simulink model "Intro2AV_FinalProjectModel_DT"  (R2024b)
settings: Solver=VariableStepAuto  StartTime=0.0  StopTime=72  RelTol=1e-3
values from neighbouring files (symbols this model uses):
  gradbp = linspace(0,totalDistance,50)    [scriptRefDataDT.m]
  thetaRefs = smooth(gradbp,thetaRef)    [scriptRefDataDT.m]
  xRef2s = smooth(gradbp,xRef2)    [scriptRefDataDT.m]
  yRef2s = smooth(gradbp,yRef2)    [scriptRefDataDT.m]
libraries: drivingvehiclecontroller x1
settings Model: Creator=lpdtd  LastModifiedBy=lpdtd

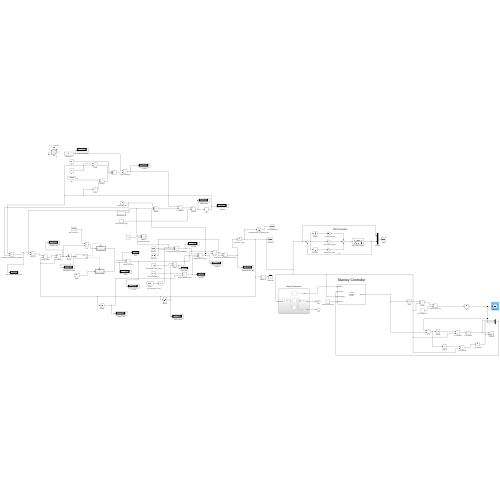
[thumbnail: Simulink's stored preview of the top-level diagram]
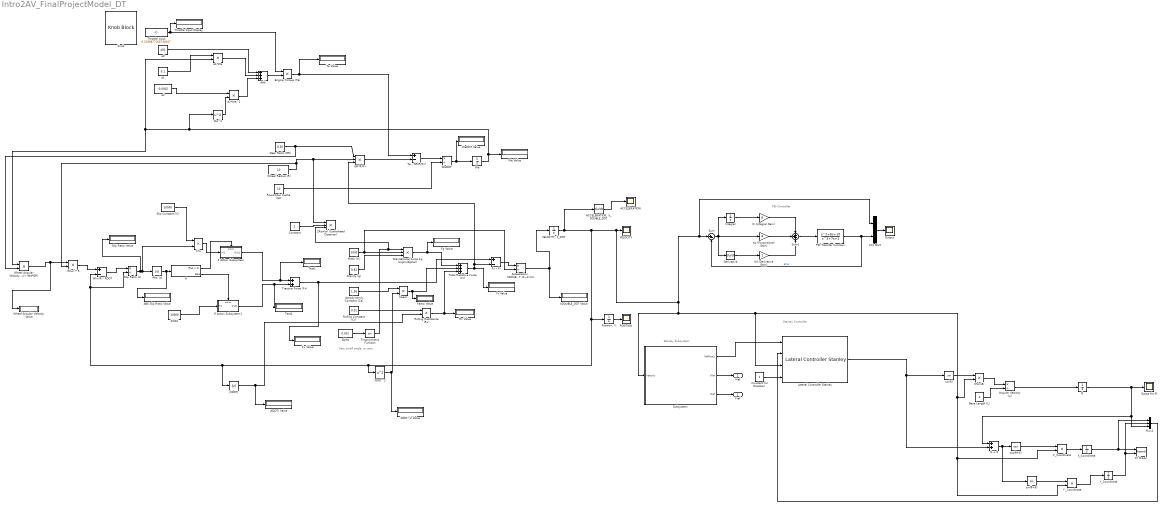
== system Intro2AV_FinalProjectModel_DT ==
  note: Stanley Controller
  note: Stanley Subsystem
  note: Very small angle, or zero.
  note: PID Controller
  2Rsin(a) (Lookahead Distance) : Product  Inputs=3
  2X1 MUX : Mux  Inputs=2
  ABS Slip Ratio Value : Display
  ACCELERATION : Scope
  "ACCELERATION, X_DOUBLE_DOT" : Derivative
  "Abs, |s|" : Abs  SaturateOnIntegerOverflow=off
  "Acceleration, XDOUBLE_DOT (Fx-Fr)/m" : Product  Inputs=*/
  Add : Sum  Inputs=+++
  Aerodynamic Constant (Ca) : Constant  Value=1.36
  Alpha : Constant  Value=0.001
  Angular Velocity (ω) : Product  Inputs=*/
  Base Length (L) : Constant  Value=4
  C*s : Product
  Constant : Constant  Value=2
  Constant for Direction : Constant
  "Derivative " : Derivative
  Engine Torque (Te) : Product
  FMAX : Constant  Value=10000
  Faero : Product
  Faero Value : Display
  Fg Value : Display
  Fr Value : Display
  Fx - Fr : Sum  Inputs=+-
  Fx Value : Display
  GR*R*Fr : Product  Inputs=3
  Gear Ratio (GR) : Constant  Value=0.35
  Gravitational Force Fg (mgsin(Alpha)) : Product  Inputs=3
  Gravity (g) : Constant  Value=9.81
  If : If  IfExpression=u1 < 1
  If Action Subsystem : Subsystem  TreatAsAtomicUnit=on
  If Action Subsystem1 : Subsystem  TreatAsAtomicUnit=on
  Integral : Integrator
  Kd (Derivative Gain) : Gain
  Ki (Integral Gain) : Gain  Gain=6
  Knob : KnobBlock  ScaleMax=1
  Kp (Porportional Gain) : Gain  Gain=4
  Lateral Controller Stanley : drivingvehiclecontroller/Lateral Controller Stanley  ModelType=Kinematic bicycle model  PositionGainF=2.5  PositionGainR=2.5  YawRateGain=0.2  DelayGain=0.2  VehicleMass=1575  Lf=1.2  Lr=1.6  TireStiffness=19000  Wheelbase=2.8  MaxSteeringAngle=35
  Mass (m) : Constant  Value=2000
  Mux2 : Mux  Inputs=3
  Output : Scope
  PID Transfer Function : TransferFcn  Numerator=[1,6,10]  Denominator=[1,0,7,1]
  POSITION : Scope
  "Position, X" : Integrator
  Powertrain Inertia (Ipt) : Constant  Value=10
  Rolling Constant (Cr) : Constant  Value=0.01
  Rolling Resistance (Rx) : Product
  Rx Value : Display
  Scope for θ : Scope
  Slip Constant (C) : Constant  Value=10000
  Slip Ratio (s) : Product  Inputs=*/
  Slip Ratio Value : Display
  Subsystem : Subsystem
  Sum : Sum  Inputs=|+-
  Sum1 : Sum  Inputs=+++
  Te - GR(R*Fr) : Sum  Inputs=+-
  Te Value : Display
  Test1 : Display
  Test2 : Display
  Throttle Input : Constant  Value=0.3199877166748047
  Throttle Input Display : Display
  Total Resistive Force (Fr) : Sum  Inputs=+++
  Tractive Force (Fx) : Sum
  Trigonometric Function : Trigonometry
  V*sin(δ) : Product
  VELOCITY : Scope
  "VELOCITY, X_DOT" : Integrator
  W(w) * R : Product
  W(w)R - XDOT : Sum  Inputs=+-
  We : Integrator  InitialCondition=100
  We Value : Display
  WeDOT : Product  Inputs=*/
  WeDOT Value : Display
  We^2 : Math  Operator=square
  Wheel Angular Velocity Value : Display
  Wheel Angular Velocity W(w) (We*GR) : Product
  Wheel Radius (R) : Constant  Value=10
  X'_Coordinate : Product
  XDOT^2 : Math  Operator=square
  XDOT^2 Value : Display
  XDOUBLE_DOT Value : Display
  XY Graph : Record  FileSettingsInternal="{\"entries\":[{\"content\":{\"excelSettings\":{\"content\":{},\"type\":\"Streamout.ExcelSettings\"}},\"type\":\"Streamout.FileSettingStorage\",\"uuid\":\"\"}],\"packageUris\":[\"http:\\/\\/schema.mathworks.com\\/mf0\\/streamout_blocks\\/R2020a\"],\"version\":\"1.0\"}"  Layout=[1 1]  SignalsInternal="{\"entries\":[{\"content\":{\"signals\":[{\"content\":{\"blockPath\":[],\"dimensions\":[1,1],\"domain\":\"\",\"lineColor\":\"#a2142f\",\"plots\":[ 1 ],\"port\":1,\"sid\":[\"\"],\"signalID\":1,\"signalName\":\"Y_Coordinate\"},\"type\":\"RecordBlkView.Signal\",\"uuid\":\"\"},{\"content\":{\"blockPath\":[],\"dimensions\":[1,1],\"domain\":\"\",\"lineColor\":\"#a2142f\",\"plots\":[ 1 ],\"port\":2,\"sid\":[\"\"],\"signalID\":2,\"signalName\":\"X_Coordinate\"},\"type\":\"RecordBlkView.Signal\",\"uuid\":\"\"}]},\"type\":\"RecordBlkView.InputSignals\",\"uuid\":\"\"}],\"packageUris\":[\"http:\\/\\/schema.mathworks.com\\/mf0\\/streamout_blocks\\/R2020a\"],\"version\":\"1.0\"}"  VisualizationBindings="{\"xyplotplugin\":{\"info\":[{\"series\":[{\"bindingParametersList\":[{\"parameter\":\"X-Axis\",\"signalID\":1,\"signalName\":\"Y_Coordinate\"},{\"parameter\":\"Y-Axis\",\"signalID\":2,\"signalName\":\"X_Coordinate\"}],\"seriesID\":0}],\"subplotID\":1}]}}"  CompatibilityTag=XY
  X_Coordinate : Integrator  InitialCondition=2.25
  Y'_Coordinate : Product
  Y_Coordinate : Integrator  InitialCondition=1.89
  a0 : Constant  Value=400
  a1 : Constant  Value=0.1
  a1*We : Product
  a2 : Constant  Value=-0.0002
  a2*We^2 : Product
  cos(θ+δ) : Trigonometry  Operator=cos
  sin(δ) : Trigonometry
  sin(θ+δ) : Trigonometry
  |XDOT| : Abs  SaturateOnIntegerOverflow=off
  |XDOT| Value : Display
  θ : Integrator  InitialCondition=0.02
  θ + δ : Sum
  Yref : Outport
  Xref : Outport  Port=2
  wires:
  a1/1 -> a1*We/1
  a2/1 -> a2*We^2/1
  We^2/1 -> a2*We^2/2
  a0/1 -> Add/1
  a1*We/1 -> Add/2
  a2*We^2/1 -> Add/3
  Add/1 -> Engine Torque (Te)/2
  Throttle Input/1 -> Engine Torque (Te)/1, Throttle Input Display/1
  "Abs, |s|"/1 -> ABS Slip Ratio Value/1, If/1
  Gear Ratio (GR)/1 -> Wheel Angular Velocity W(w) (We*GR)/2, GR*R*Fr/1
  Wheel Radius (R)/1 -> 2Rsin(a) (Lookahead Distance)/1, GR*R*Fr/2, W(w) * R/2
  W(w) * R/1 -> W(w)R - XDOT/1
  W(w)R - XDOT/1 -> Slip Ratio (s)/1
  Slip Ratio (s)/1 -> Slip Ratio Value/1, C*s/2, "Abs, |s|"/1
  Slip Constant (C)/1 -> C*s/1
  Mass (m)/1 -> "Acceleration, XDOUBLE_DOT (Fx-Fr)/m"/2, Gravitational Force Fg (mgsin(Alpha))/2
  Gravity (g)/1 -> Gravitational Force Fg (mgsin(Alpha))/3
  Trigonometric Function/1 -> 2Rsin(a) (Lookahead Distance)/3, Gravitational Force Fg (mgsin(Alpha))/1
  XDOT^2/1 -> XDOT^2 Value/1, Faero/2
  Aerodynamic Constant (Ca)/1 -> Faero/1
  |XDOT|/1 -> |XDOT| Value/1, Rolling Resistance (Rx)/2
  Rolling Constant (Cr)/1 -> Rolling Resistance (Rx)/1
  Rolling Resistance (Rx)/1 -> Rx Value/1, Total Resistive Force (Fr)/3
  Faero/1 -> Faero Value/1, Total Resistive Force (Fr)/2
  Gravitational Force Fg (mgsin(Alpha))/1 -> Fg Value/1, Total Resistive Force (Fr)/1
  Total Resistive Force (Fr)/1 -> Fr Value/1, Fx - Fr/2, GR*R*Fr/3
  GR*R*Fr/1 -> Te - GR(R*Fr)/2
  Te - GR(R*Fr)/1 -> WeDOT/1
  Powertrain Inertia (Ipt)/1 -> WeDOT/2
  WeDOT/1 -> WeDOT Value/1, We/1
  Tractive Force (Fx)/1 -> Fx Value/1, Fx - Fr/1
  Fx - Fr/1 -> "Acceleration, XDOUBLE_DOT (Fx-Fr)/m"/1
  "Acceleration, XDOUBLE_DOT (Fx-Fr)/m"/1 -> "VELOCITY, X_DOT"/1, XDOUBLE_DOT Value/1
  "Position, X"/1 -> POSITION/1
  If/1 -> If Action Subsystem/Action
  If/2 -> If Action Subsystem1/Action
  C*s/1 -> If Action Subsystem/1(In1)
  If Action Subsystem/1(Out1) -> Test1/1, Tractive Force (Fx)/1
  FMAX/1 -> If Action Subsystem1/1(In1)
  If Action Subsystem1/1(Out1) -> Test2/1, Tractive Force (Fx)/2
  We/1 -> We Value/1, Wheel Angular Velocity W(w) (We*GR)/1, a1*We/2, We^2/1
  Engine Torque (Te)/1 -> Te Value/1, Te - GR(R*Fr)/1
  Wheel Angular Velocity W(w) (We*GR)/1 -> Wheel Angular Velocity Value/1, W(w) * R/1
  Alpha/1 -> Trigonometric Function/1
  Constant/1 -> 2Rsin(a) (Lookahead Distance)/2
  Kd (Derivative Gain)/1 -> Sum1/3
  Sum1/1 -> PID Transfer Function/1
  "Derivative "/1 -> Kd (Derivative Gain)/1
  Integral/1 -> Ki (Integral Gain)/1
  Ki (Integral Gain)/1 -> Sum1/1
  Kp (Porportional Gain)/1 -> Sum1/2
  PID Transfer Function/1 -> Sum/2, 2X1 MUX/2  "Error"
  2X1 MUX/1 -> Output/1
  Sum/1 -> "Derivative "/1, Integral/1, Kp (Porportional Gain)/1
  X_Coordinate/1 -> Mux2/1, XY Graph/1
  Y'_Coordinate/1 -> Y_Coordinate/1
  X'_Coordinate/1 -> X_Coordinate/1
  Lateral Controller Stanley/1 -> θ + δ/2, sin(δ)/1
  Base Length (L)/1 -> Angular Velocity (ω)/2
  Mux2/1 -> Lateral Controller Stanley/2
  "VELOCITY, X_DOT"/1 -> "ACCELERATION, X_DOUBLE_DOT"/1, "Position, X"/1, XDOT^2/1, Slip Ratio (s)/2, W(w)R - XDOT/2, |XDOT|/1, VELOCITY/1, 2X1 MUX/1, Sum/1, Y'_Coordinate/2, X'_Coordinate/2, V*sin(δ)/2, Lateral Controller Stanley/3, Subsystem/1(Velocity)
  θ/1 -> Scope for θ/1, θ + δ/1, Mux2/3
  θ + δ/1 -> sin(θ+δ)/1, cos(θ+δ)/1
  sin(δ)/1 -> V*sin(δ)/1
  Angular Velocity (ω)/1 -> θ/1
  Constant for Direction/1 -> Lateral Controller Stanley/4
  V*sin(δ)/1 -> Angular Velocity (ω)/1
  sin(θ+δ)/1 -> Y'_Coordinate/1
  cos(θ+δ)/1 -> X'_Coordinate/1
  "ACCELERATION, X_DOUBLE_DOT"/1 -> ACCELERATION/1
  Subsystem/3(YRef) -> Yref/1
  Subsystem/1(RefPose1) -> Lateral Controller Stanley/1
  Subsystem/2(XRef) -> Xref/1
  Y_Coordinate/1 -> XY Graph/2, Mux2/2

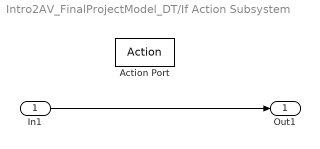
== system Intro2AV_FinalProjectModel_DT/If Action Subsystem ==
  In1 : Inport
  Action Port : ActionPort  ActionPortLabel=if(u1 < 1)
  Out1 : Outport
  wires:
  In1/1 -> Out1/1

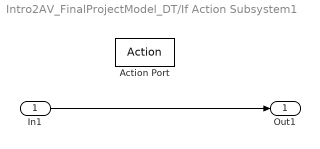
== system Intro2AV_FinalProjectModel_DT/If Action Subsystem1 ==
  In1 : Inport
  Action Port : ActionPort  ActionPortLabel=else
  Out1 : Outport
  wires:
  In1/1 -> Out1/1

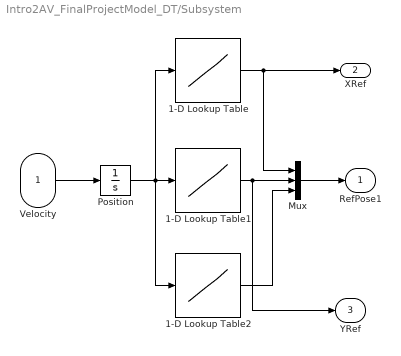
== system Intro2AV_FinalProjectModel_DT/Subsystem ==
  Velocity : Inport
  1-D Lookup Table : Lookup_n-D  NumberOfTableDimensions=1  BreakpointsForDimension1=gradbp  Table=xRef2s  InternalRulePriority=Speed  RndMeth=Simplest
  1-D Lookup Table1 : Lookup_n-D  NumberOfTableDimensions=1  BreakpointsForDimension1=gradbp  Table=yRef2s  InternalRulePriority=Speed  RndMeth=Simplest
  1-D Lookup Table2 : Lookup_n-D  NumberOfTableDimensions=1  BreakpointsForDimension1=gradbp  Table=thetaRefs  InternalRulePriority=Speed  RndMeth=Simplest
  Mux : Mux  Inputs=3
  Position : Integrator
  RefPose1 : Outport
  XRef : Outport  Port=2
  YRef : Outport  Port=3
  wires:
  Velocity/1 -> Position/1
  Position/1 -> 1-D Lookup Table2/1, 1-D Lookup Table1/1, 1-D Lookup Table/1
  1-D Lookup Table/1 -> Mux/1, XRef/1
  1-D Lookup Table2/1 -> Mux/3
  Mux/1 -> RefPose1/1
  1-D Lookup Table1/1 -> Mux/2, YRef/1
